simulink model "Part4_5_WLTP"  (R2019b)
settings: Solver=FixedStepAuto  StartTime=0.0  StopTime=1800  FixedStep=0.1  RelTol=1e-3
model workspace (MAT data in the model file):
  A = 2.2
  Achsgetriebewirkungsgrad = 0.95
  E_ges = 60
  F_Reib = 40
  Getriebewirkungsgrad = 0.95
  M_gen_max = -2382
  MaxBremskraft = 7005.88
  Maxdrehmoment = 3460
  Pho = 1.225
  SOC_Init = 0.8
  c = 0.3
  eta1 = 0.95
  h = 0.5
  i_ag = 0.95
  i_g = 0.95
  l = 1.3
  lambda = 1.05
  miu = 1
  rdy = 0.34
values from neighbouring files (symbols this model uses):
  F_Roll = 125.568    [EBV_Par.mat]
  full_load_M_gen = [nan -147.541722889 -211.594901974 -211.605758729 -211.377214201 -211.387947431 -211.398597277 -211.40916374 -211.419646819 -211.430046515 -211.440362826 -211.450595754 ... (79 elements, 1x79)]    [EBV_Par.mat]
  full_load_M_mot = [307.16713761 307.16713761 307.15125253 307.13548852 307.119845585 307.104323723 307.088922934 307.073643217 307.058484574 307.043447004 307.028530508 307.013735084 ... (79 elements, 1x79)]    [EBV_Par.mat]
  full_load_n = [0 200 400 600 800 1000 1200 1400 1600 1800 2000 2200 ... (79 elements, 1x79)]    [EBV_Par.mat]
  g = 9.81    [EBV_Par.mat]
  iag = 4    [EBV_Par.mat]
  ig = 3.12    [EBV_Par.mat]
  m = 1600    [EBV_Par.mat]
  M_loss_gen_grid = [3.32247584497 3.32247584497 1.76322338006 1.23912671725 0.984972087819 0.841812429894 0.753172614648 0.695924215073 0.655195160155 0.6126512242 0.552159885143 0.497873417445 ... (2943 elements, 27x109)]    [EBV_Par.mat]
  M_loss_mot_grid = [2.25037598951 2.25037598951 1.16187270775 0.818485589561 0.655488271287 0.566699700914 0.515063220158 0.480627768817 0.45851815067 0.444966043153 0.436284256227 0.436981398972 ... (2943 elements, 27x109)]    [EBV_Par.mat]
  M_lut = [0 2.86111111111 5.72222222222 8.58333333333 11.4444444444 14.3055555556 17.1666666667 20.0277777778 22.8888888889 25.75 28.6111111111 31.4722222222 ... (109 elements, 1x109)]    [EBV_Par.mat]
  n_lut = [0 615.384615385 1230.76923077 1846.15384615 2461.53846154 3076.92307692 3692.30769231 4307.69230769 4923.07692308 5538.46153846 6153.84615385 6769.23076923 ... (27 elements, 27x1)]    [EBV_Par.mat]
libraries: simulink x3
settings Model: Creator=kingtakepc  LastModifiedBy=kingtakepc
settings DebuggingCC: SFMachineParentedDataDiag=error

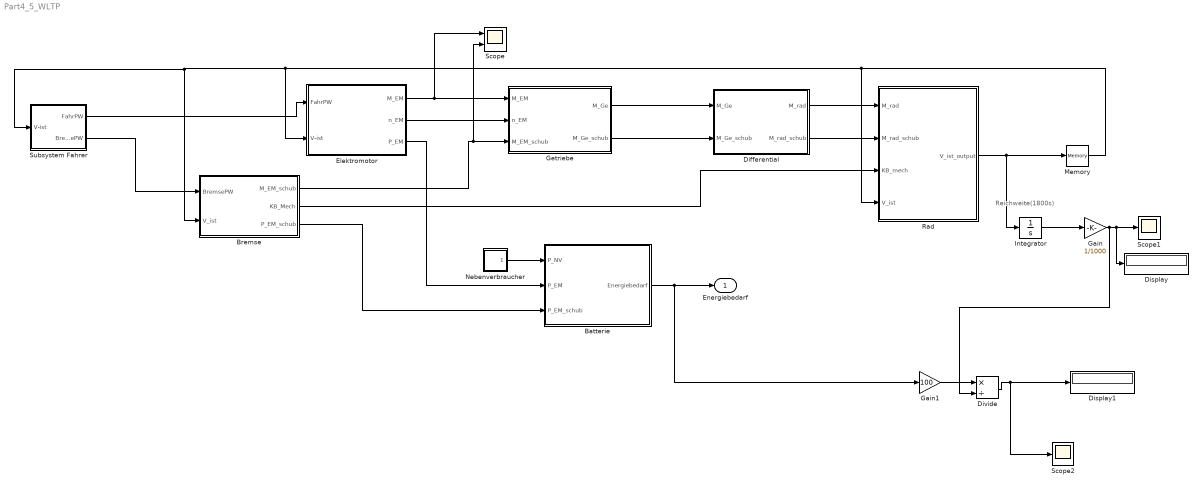
== system Part4_5_WLTP ==
  note: Reichweite(1800s)
  Batterie : Subsystem
  Bremse : Subsystem
  Differential : Subsystem
  Display : Display
  Display1 : Display
  Divide : Product  Inputs=*/
  Elektromotor : Subsystem
  Gain : Gain  Gain=1/1000
  Gain1 : Gain  Gain=100
  Getriebe : Subsystem
  Integrator : Integrator
  Memory : Memory
  Nebenverbraucher : Subsystem
  Rad : Subsystem
  Scope : Scope  NumInputPorts=2
  Scope1 : Scope
  Scope2 : Scope
  Subsystem Fahrer : Subsystem
  Energiebedarf : Outport
  wires:
  Getriebe/1(M_Ge) -> Differential/1(M_Ge)
  Differential/1(M_rad) -> Rad/1(M_rad)
  Nebenverbraucher/1(P_NV) -> Batterie/1(P_NV)
  Batterie/1(Energiebedarf) -> Gain1/1, Energiebedarf/1
  Getriebe/2(M_Ge_schub) -> Differential/2(M_Ge_schub)
  Differential/2(M_rad_schub) -> Rad/2(M_rad_schub)
  Elektromotor/1(M_EM) -> Scope/1, Getriebe/1(M_EM)
  Elektromotor/2(n_EM) -> Getriebe/2(n_EM)
  Elektromotor/3(P_EM) -> Batterie/2(P_EM)
  Bremse/3(P_EM_schub) -> Batterie/3(P_EM_schub)
  Bremse/1(M_EM_schub) -> Scope/2, Getriebe/3(M_EM_schub)
  Bremse/2(KB_Mech) -> Rad/3(KB_mech)
  Rad/1(V_ist_output) -> Integrator/1, Memory/1
  Memory/1 -> Rad/4(V_ist), Elektromotor/2(V-ist), Subsystem Fahrer/1(V-ist), Bremse/2(V_ist)
  Subsystem Fahrer/2(BremsePW) -> Bremse/1(BremsePW)
  Subsystem Fahrer/1(FahrPW) -> Elektromotor/1(FahrPW)
  Integrator/1 -> Gain/1
  Gain/1 -> Divide/2, Display/1, Scope1/1
  Gain1/1 -> Divide/1
  Divide/1 -> Scope2/1, Display1/1

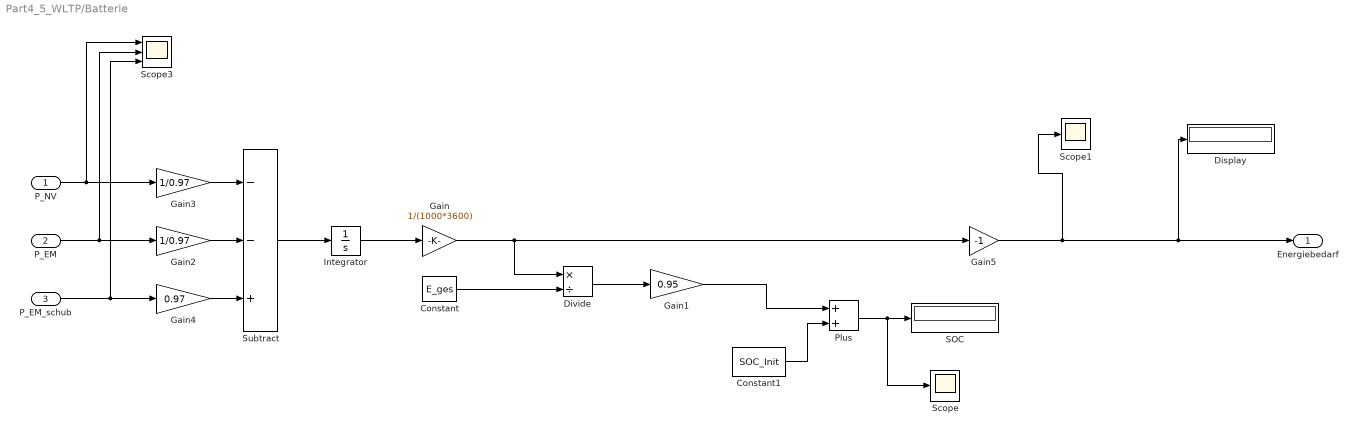
== system Part4_5_WLTP/Batterie ==
  P_NV : Inport
  P_EM : Inport  Port=2
  P_EM_schub : Inport  Port=3
  Constant : Constant  Value=E_ges
  Constant1 : Constant  Value=SOC_Init
  Display : Display
  Divide : Product  Inputs=*/
  Gain : Gain  Gain=1/(1000*3600)
  Gain1 : Gain  Gain=0.95
  Gain2 : Gain  Gain=1/0.97
  Gain3 : Gain  Gain=1/0.97
  Gain4 : Gain  Gain=0.97
  Gain5 : Gain  Gain=-1
  Integrator : Integrator
  Plus : Sum
  SOC : Display
  Scope : Scope
  Scope1 : Scope
  Scope3 : Scope  NumInputPorts=3
  Subtract : Sum  Inputs=--+
  Energiebedarf : Outport
  wires:
  P_NV/1 -> Scope3/1, Gain3/1
  P_EM/1 -> Scope3/2, Gain2/1
  P_EM_schub/1 -> Scope3/3, Gain4/1
  Subtract/1 -> Integrator/1
  Integrator/1 -> Gain/1
  Constant/1 -> Divide/2
  Divide/1 -> Gain1/1
  Constant1/1 -> Plus/2
  Gain2/1 -> Subtract/2
  Gain3/1 -> Subtract/1
  Gain4/1 -> Subtract/3
  Gain1/1 -> Plus/1
  Plus/1 -> Scope/1, SOC/1
  Gain/1 -> Divide/1, Gain5/1
  Gain5/1 -> Scope1/1, Display/1, Energiebedarf/1

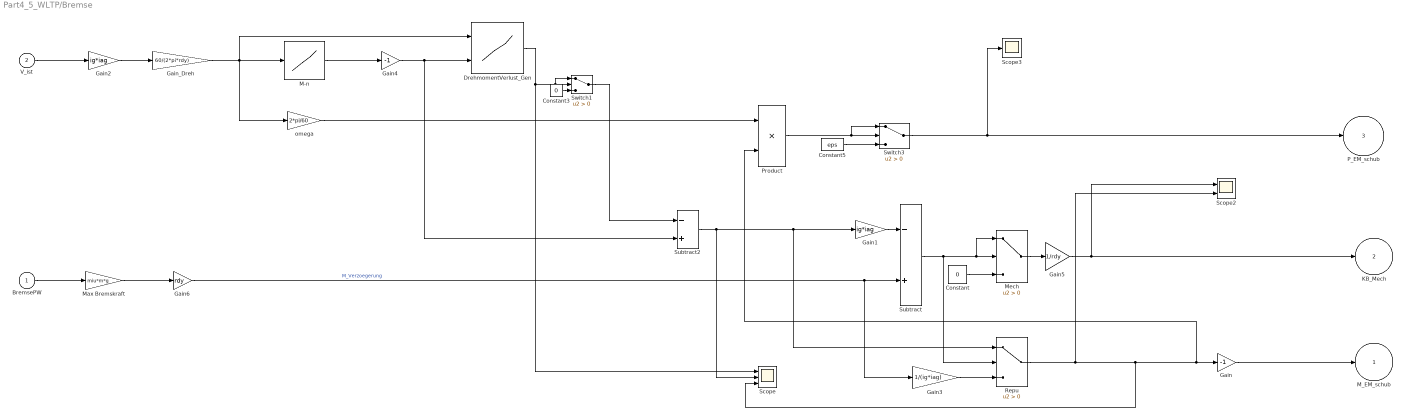
== system Part4_5_WLTP/Bremse ==
  BremsePW : Inport
  V_ist : Inport  Port=2
  Constant : Constant  Value=0
  Constant3 : Constant  Value=0
  Constant5 : Constant  Value=eps
  DrehmomentVerlust_Gen : Lookup_n-D  BreakpointsForDimension1=n_lut  BreakpointsForDimension2=M_lut  Table=M_loss_gen_grid  InternalRulePriority=Speed  RndMeth=Simplest  InputSameDT=on
  Gain : Gain  Gain=-1
  Gain1 : Gain  Gain=ig*iag
  Gain2 : Gain  Gain=ig*iag
  Gain3 : Gain  Gain=1/(ig*iag)
  Gain4 : Gain  Gain=-1
  Gain5 : Gain  Gain=1/rdy
  Gain6 : Gain  Gain=rdy
  Gain_Dreh : Gain  Gain=60/(2*pi*rdy)
  "M-n " : Lookup_n-D  NumberOfTableDimensions=1  BreakpointsForDimension1=full_load_n  Table=full_load_M_gen  InternalRulePriority=Speed  RndMeth=Simplest  InputSameDT=on
  Max Bremskraft : Gain  Gain=miu*m*g
  Mech : Switch  Criteria=u2 > Threshold
  Product : Product
  Repu : Switch  Criteria=u2 > Threshold
  Scope : Scope  NumInputPorts=3
  Scope2 : Scope  NumInputPorts=2
  Scope3 : Scope
  Subtract : Sum  Inputs=-+
  Subtract2 : Sum  Inputs=-+
  Switch1 : Switch  Criteria=u2 > Threshold
  Switch3 : Switch  Criteria=u2 > Threshold
  omega : Gain  Gain=2*pi/60
  M_EM_schub : Outport
  KB_Mech : Outport  Port=2
  P_EM_schub : Outport  Port=3
  wires:
  V_ist/1 -> Gain2/1
  Gain2/1 -> Gain_Dreh/1
  Gain_Dreh/1 -> DrehmomentVerlust_Gen/1, omega/1, "M-n "/1
  omega/1 -> Product/1
  DrehmomentVerlust_Gen/1 -> Scope/1, Switch1/1, Switch1/2
  Constant3/1 -> Switch1/3
  Switch1/1 -> Subtract2/1
  Product/1 -> Switch3/1, Switch3/2
  Subtract2/1 -> Scope/2, Repu/1, Gain1/1
  Constant5/1 -> Switch3/3
  BremsePW/1 -> Max Bremskraft/1
  Max Bremskraft/1 -> Gain6/1
  Gain6/1 -> Gain3/1, Subtract/2  "M_Verzoegerung"
  Subtract/1 -> Repu/2, Mech/1, Mech/2
  Gain1/1 -> Subtract/1
  Mech/1 -> Gain5/1
  Constant/1 -> Mech/3
  Gain3/1 -> Repu/3
  Repu/1 -> Scope2/2, Scope/3, Product/2, Gain/1
  Switch3/1 -> Scope3/1, P_EM_schub/1
  Gain/1 -> M_EM_schub/1
  "M-n "/1 -> Gain4/1
  Gain4/1 -> Subtract2/2, DrehmomentVerlust_Gen/2
  Gain5/1 -> Scope2/1, KB_Mech/1

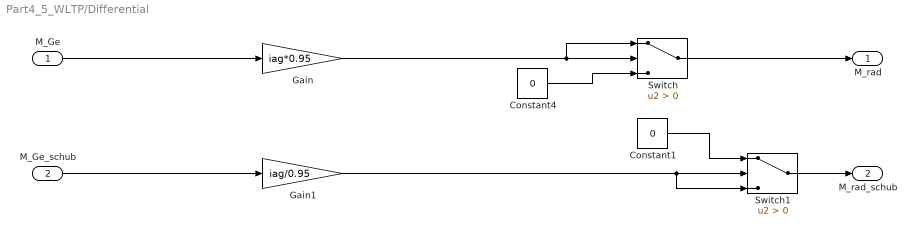
== system Part4_5_WLTP/Differential ==
  M_Ge : Inport
  M_Ge_schub : Inport  Port=2
  Constant1 : Constant  Value=0
  Constant4 : Constant  Value=0
  Gain : Gain  Gain=iag*0.95
  Gain1 : Gain  Gain=iag/0.95
  Switch : Switch  Criteria=u2 > Threshold
  Switch1 : Switch  Criteria=u2 > Threshold
  M_rad : Outport
  M_rad_schub : Outport  Port=2
  wires:
  M_Ge/1 -> Gain/1
  M_Ge_schub/1 -> Gain1/1
  Switch/1 -> M_rad/1
  Gain/1 -> Switch/1, Switch/2
  Constant4/1 -> Switch/3
  Switch1/1 -> M_rad_schub/1
  Gain1/1 -> Switch1/3, Switch1/2
  Constant1/1 -> Switch1/1

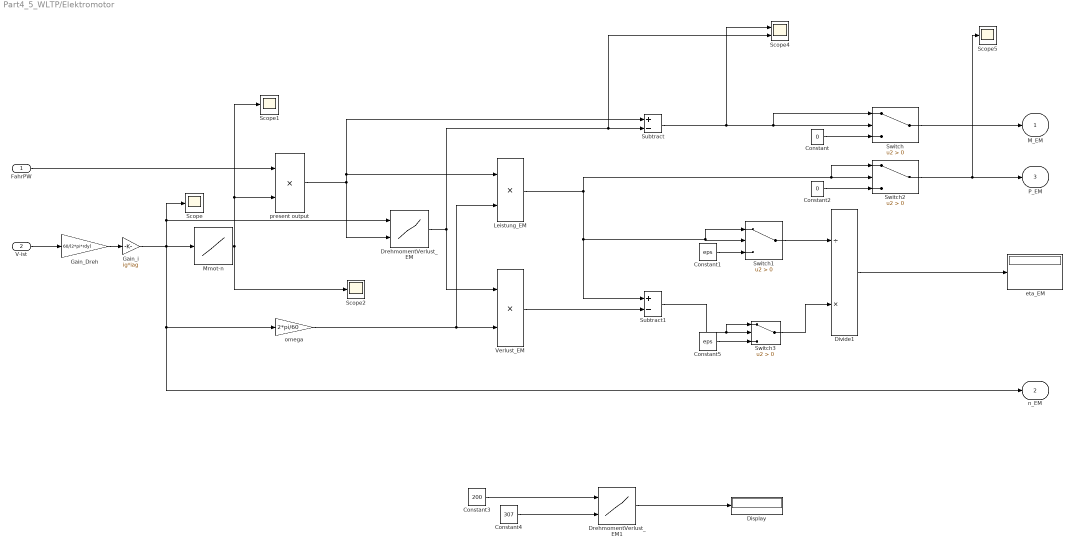
== system Part4_5_WLTP/Elektromotor ==
  FahrPW : Inport
  V-ist : Inport  Port=2
  " Leistung_EM" : Product
  Constant : Constant  Value=0
  Constant1 : Constant  Value=eps
  Constant2 : Constant  Value=0
  Constant3 : Constant  Value=200
  Constant4 : Constant  Value=307
  Constant5 : Constant  Value=eps
  Display : Display
  Divide1 : Product  Inputs=/*
  DrehmomentVerlust_EM : Lookup_n-D  BreakpointsForDimension1=n_lut  BreakpointsForDimension2=M_lut  Table=M_loss_mot_grid  InternalRulePriority=Speed  RndMeth=Simplest  InputSameDT=on
  DrehmomentVerlust_EM1 : Lookup_n-D  BreakpointsForDimension1=n_lut  BreakpointsForDimension2=M_lut  Table=M_loss_mot_grid  InternalRulePriority=Speed  RndMeth=Simplest  InputSameDT=on
  Gain_Dreh : Gain  Gain=60/(2*pi*rdy)
  Gain_i : Gain  Gain=ig*iag
  Mmot-n : Lookup_n-D  NumberOfTableDimensions=1  BreakpointsForDimension1=full_load_n  Table=full_load_M_mot  InternalRulePriority=Speed  RndMeth=Simplest  InputSameDT=on
  Scope{,1..2,5} (4 alike) : Scope
  Scope4 : Scope  NumInputPorts=2
  Subtract : Sum  Inputs=+-
  Subtract1 : Sum  Inputs=+-
  Switch{,1..3} (4 alike) : Switch  Criteria=u2 > Threshold
  Verlust_EM : Product
  eta_EM : Display
  omega : Gain  Gain=2*pi/60
  present output : Product
  M_EM : Outport
  n_EM : Outport  Port=2
  P_EM : Outport  Port=3
  wires:
  FahrPW/1 -> present output/1
  V-ist/1 -> Gain_Dreh/1
  Gain_Dreh/1 -> Gain_i/1
  Gain_i/1 -> Scope/1, DrehmomentVerlust_EM/1, n_EM/1, omega/1, Mmot-n/1
  Mmot-n/1 -> Scope1/1, present output/2, Scope2/1
  DrehmomentVerlust_EM/1 -> Verlust_EM/1, Scope4/2, Subtract/2
  Subtract/1 -> Scope4/1, Switch/1, Switch/2
  Constant/1 -> Switch/3
  present output/1 -> DrehmomentVerlust_EM/2, Subtract/1, " Leistung_EM"/1
  omega/1 -> " Leistung_EM"/2, Verlust_EM/2
  " Leistung_EM"/1 -> Switch2/1, Switch2/2, Subtract1/1, Switch1/1, Switch1/2
  Switch1/1 -> Divide1/1
  Constant1/1 -> Switch1/3
  Divide1/1 -> eta_EM/1
  Constant2/1 -> Switch2/3
  Switch2/1 -> Scope5/1, P_EM/1
  Switch/1 -> M_EM/1
  Subtract1/1 -> Switch3/1, Switch3/2
  Verlust_EM/1 -> Subtract1/2
  Constant3/1 -> DrehmomentVerlust_EM1/1
  DrehmomentVerlust_EM1/1 -> Display/1
  Constant4/1 -> DrehmomentVerlust_EM1/2
  Constant5/1 -> Switch3/3
  Switch3/1 -> Divide1/2

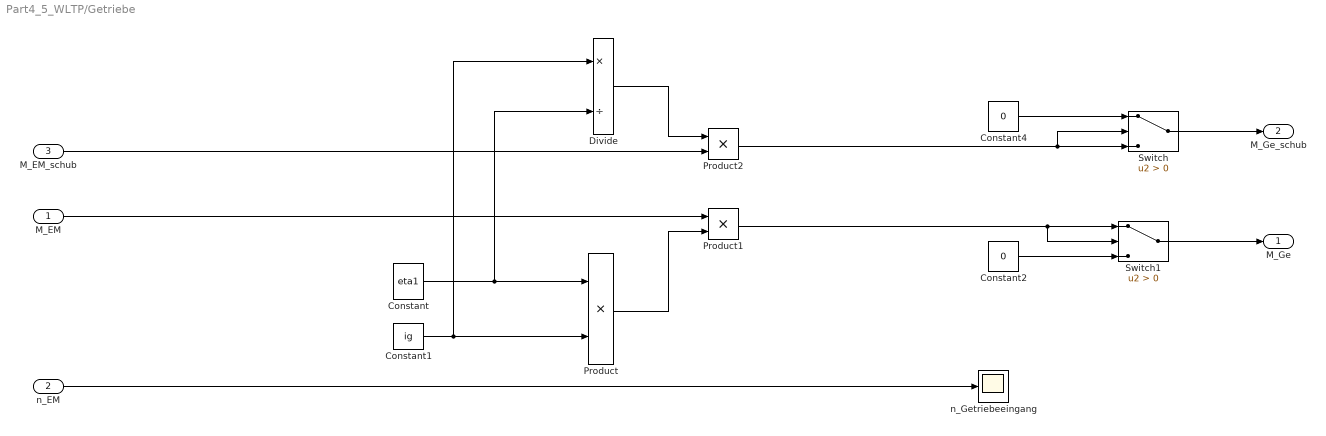
== system Part4_5_WLTP/Getriebe ==
  M_EM : Inport
  n_EM : Inport  Port=2
  M_EM_schub : Inport  Port=3
  Constant : Constant  Value=eta1
  Constant1 : Constant  Value=ig
  Constant2 : Constant  Value=0
  Constant4 : Constant  Value=0
  Divide : Product  Inputs=*/
  Product : Product
  Product1 : Product
  Product2 : Product
  Switch : Switch  Criteria=u2 > Threshold
  Switch1 : Switch  Criteria=u2 > Threshold
  n_Getriebeeingang : Scope
  M_Ge : Outport
  M_Ge_schub : Outport  Port=2
  wires:
  Constant1/1 -> Divide/1, Product/2
  M_EM/1 -> Product1/1
  Constant/1 -> Divide/2, Product/1
  Product/1 -> Product1/2
  n_EM/1 -> n_Getriebeeingang/1
  M_EM_schub/1 -> Product2/2
  Divide/1 -> Product2/1
  Switch/1 -> M_Ge_schub/1
  Product2/1 -> Switch/2, Switch/3
  Constant4/1 -> Switch/1
  Switch1/1 -> M_Ge/1
  Product1/1 -> Switch1/2, Switch1/1
  Constant2/1 -> Switch1/3

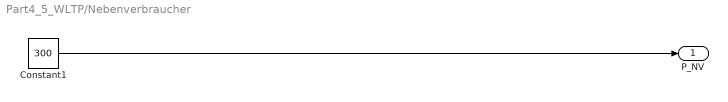
== system Part4_5_WLTP/Nebenverbraucher ==
  Constant1 : Constant  Value=300
  P_NV : Outport
  wires:
  Constant1/1 -> P_NV/1

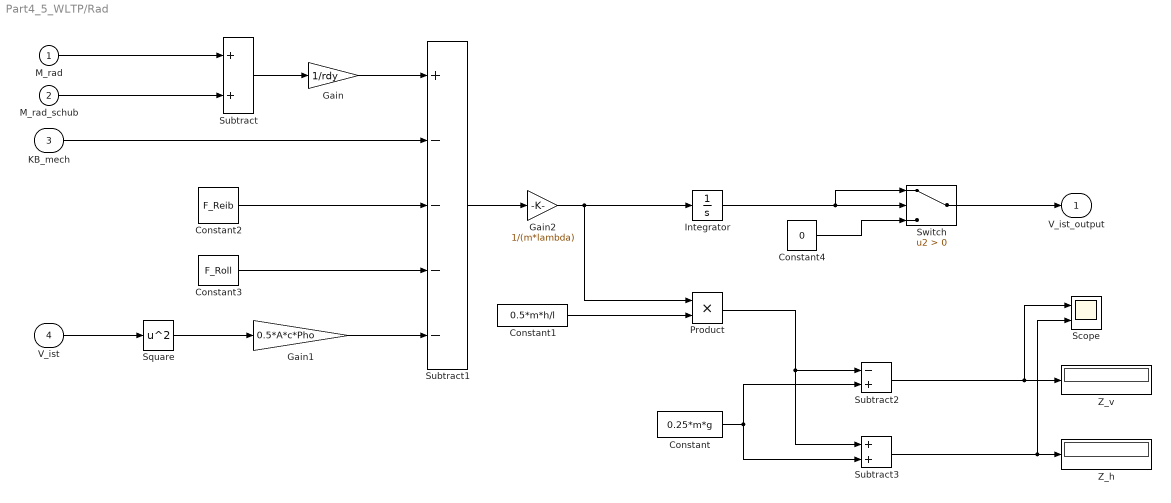
== system Part4_5_WLTP/Rad ==
  M_rad : Inport
  M_rad_schub : Inport  Port=2
  KB_mech : Inport  Port=3
  V_ist : Inport  Port=4
  Constant : Constant  Value=0.25*m*g
  Constant1 : Constant  Value=0.5*m*h/l
  Constant2 : Constant  Value=F_Reib
  Constant3 : Constant  Value=F_Roll
  Constant4 : Constant  Value=0
  Gain : Gain  Gain=1/rdy
  Gain1 : Gain  Gain=0.5*A*c*Pho
  Gain2 : Gain  Gain=1/(m*lambda)
  Integrator : Integrator
  Product : Product
  Scope : Scope  NumInputPorts=2
  Square : Math  Operator=square  SaturateOnIntegerOverflow=on
  Subtract : Sum
  Subtract1 : Sum  Inputs=+----
  Subtract2 : Sum  Inputs=-+
  Subtract3 : Sum
  Switch : Switch  Criteria=u2 > Threshold
  Z_h : Display
  Z_v : Display
  V_ist_output : Outport
  wires:
  M_rad/1 -> Subtract/1
  M_rad_schub/1 -> Subtract/2
  Subtract/1 -> Gain/1
  Gain/1 -> Subtract1/1
  KB_mech/1 -> Subtract1/2
  Constant2/1 -> Subtract1/3
  Constant3/1 -> Subtract1/4
  V_ist/1 -> Square/1
  Square/1 -> Gain1/1
  Gain1/1 -> Subtract1/5
  Subtract1/1 -> Gain2/1
  Gain2/1 -> Product/1, Integrator/1
  Integrator/1 -> Switch/1, Switch/2
  Constant1/1 -> Product/2
  Subtract2/1 -> Scope/1, Z_v/1
  Subtract3/1 -> Scope/2, Z_h/1
  Product/1 -> Subtract3/1, Subtract2/1
  Constant/1 -> Subtract3/2, Subtract2/2
  Constant4/1 -> Switch/3
  Switch/1 -> V_ist_output/1

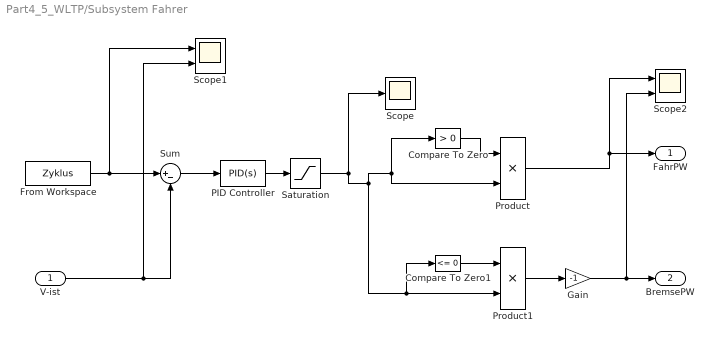
== system Part4_5_WLTP/Subsystem Fahrer ==
  V-ist : Inport
  Compare To Zero : simulink/Logic and Bit Operations/Compare To Zero  relop=>  OutDataTypeStr=boolean
  Compare To Zero1 : simulink/Logic and Bit Operations/Compare To Zero  relop=<=  OutDataTypeStr=boolean
  From Workspace : FromWorkspace  VariableName=Zyklus
  Gain : Gain  Gain=-1
  PID Controller : simulink/Continuous/PID Controller  Controller=PID  Form=Parallel  TimeDomain=Continuous-time  SampleTime=-1  IntegratorMethod=Forward Euler  FilterMethod=Forward Euler  ControllerParametersSource=internal  P=0.5  I=0.001  D=0  UseFilter=on  N=100  TunerSelectOption=Transfer Function Based (PID Tuner App)  InitialConditionSource=internal  InitialConditionForIntegrator=0  InitialConditionForFilter=0  DifferentiatorICPrevScaledInput=0  ExternalReset=none  TrackingMode=off  Kt=1  LimitOutput=off  UpperSaturationLimit=inf  LowerSaturationLimit=-inf  LinearizeAsGain=on  AntiWindupMode=none  Kb=1  POutMin=[]  POutMax=[]  IOutMin=[]  IOutMax=[]  DOutMin=[]  DOutMax=[]  NOutMin=[]  NOutMax=[]  SumOutMin=[]  SumOutMax=[]  SaturationOutMin=[]  SaturationOutMax=[]  PParamMin=[]  PParamMax=[]  IParamMin=[]  IParamMax=[]  DParamMin=[]  DParamMax=[]  NParamMin=[]  NParamMax=[]  KbParamMin=[]  KbParamMax=[]  KtParamMin=[]  KtParamMax=[]  KbOutMin=[]  KbOutMax=[]  KtOutMin=[]  KtOutMax=[]  IntegratorOutMin=[]  IntegratorOutMax=[]  FilterOutMin=[]  FilterOutMax=[]  SumI1OutMin=[]  SumI1OutMax=[]  SumI2OutMin=[]  SumI2OutMax=[]  SumI3OutMin=[]  SumI3OutMax=[]  SumI4OutMin=[]  SumI4OutMax=[]  SumDOutMin=[]  SumDOutMax=[]  DifferentiatorOutMin=[]  DifferentiatorOutMax=[]  FilterDiffOutCoefMin=[]  FilterDiffOutCoefMax=[]  ReciprocalOutMin=[]  ReciprocalOutMax=[]  SumDenOutMin=[]  SumDenOutMax=[]  SumNumOutMin=[]  SumNumOutMax=[]  DivideOutMin=[]  DivideOutMax=[]  IntegratorContinuousStateAttributes=''  IntegratorStateMustResolveToSignalObject=off  IntegratorRTWStateStorageClass=Auto  FilterContinuousStateAttributes=''  FilterStateMustResolveToSignalObject=off  FilterRTWStateStorageClass=Auto  ParallelPVariant=InternalParameters  IdealPVariant=Disabled  IVariant=InternalParameters  DVariant=InternalParameters  IntegratorVariant=Continuous  SatVariant=Disabled  AWVariant=Passthrough  PCopyVariant=Disabled  TRVariant=Disabled  FdbkBlocksVariant=Forward  IdealPFdbkVariant=Disabled  SatFdbkVariant=Disabled  DerivativeFilterVariant=ContFilter  NVariant=InternalParameters  NCopyVariant=Disabled  FilterICVariant=InternalICsFilter  IntegratorICVariant=InternalICs  ExternalResetVariant=Disabled  TRSumVariant=Passthrough  SumFdbkVariant=Disabled  SumVariant=Sum_PID
  Product : Product
  Product1 : Product
  Saturation : Saturate  UpperLimit=1  LowerLimit=-1
  Scope : Scope
  Scope1 : Scope  NumInputPorts=2
  Scope2 : Scope  NumInputPorts=2
  Sum : Sum  Inputs=|+-
  FahrPW : Outport
  BremsePW : Outport  Port=2
  wires:
  V-ist/1 -> Scope1/2, Sum/2
  From Workspace/1 -> Scope1/1, Sum/1
  Sum/1 -> PID Controller/1
  Saturation/1 -> Compare To Zero/1, Product/2, Compare To Zero1/1, Product1/2, Scope/1
  Product/1 -> FahrPW/1, Scope2/1
  Gain/1 -> Scope2/2, BremsePW/1
  PID Controller/1 -> Saturation/1
  Compare To Zero/1 -> Product/1
  Compare To Zero1/1 -> Product1/1
  Product1/1 -> Gain/1
